simulink model "Block_Diagram_SimulinkNo1"  (R2023b)
settings: Solver=VariableStepAuto  StartTime=0.0  StopTime=20  RelTol=1e-3
values from neighbouring files (symbols this model uses):
  G1_den = [1 0 0]    [Block_DiagramNo1.m]    (also in Block_DiagramNo2.m; CSE_Block_DiagramNo2.m)
  G1_num = [0 0 1]    [Block_DiagramNo1.m]    (also in Block_DiagramNo2.m = [0 1]; CSE_Block_DiagramNo2.m = [0 1])
  G2_den = [1 1]    [Block_DiagramNo1.m]    (also in Block_DiagramNo2.m; CSE_Block_DiagramNo2.m)
  G2_num = [0 0 1]    [Block_DiagramNo1.m]    (also in Block_DiagramNo2.m = [0 1]; CSE_Block_DiagramNo2.m = [0 1])
  G3_den = [1 0]    [Block_DiagramNo1.m]    (also in Block_DiagramNo2.m; CSE_Block_DiagramNo2.m)
  G3_num = [0 1]    [Block_DiagramNo1.m]    (also in Block_DiagramNo2.m; CSE_Block_DiagramNo2.m)
  H1_den = [1 0]    [Block_DiagramNo1.m]    (also in Block_DiagramNo2.m; CSE_Block_DiagramNo2.m)
  H1_num = [0 1]    [Block_DiagramNo1.m]    (also in Block_DiagramNo2.m; CSE_Block_DiagramNo2.m)
  H2_den = [1 -1]    [Block_DiagramNo1.m]    (also in Block_DiagramNo2.m; CSE_Block_DiagramNo2.m)
  H2_num = [0 1]    [Block_DiagramNo1.m]    (also in Block_DiagramNo2.m; CSE_Block_DiagramNo2.m)
  H3_den = [1 -2]    [Block_DiagramNo1.m]    (also in Block_DiagramNo2.m; CSE_Block_DiagramNo2.m)
  H3_num = [0 1]    [Block_DiagramNo1.m]    (also in Block_DiagramNo2.m; CSE_Block_DiagramNo2.m)
  TF_reduced_den = conv(A_den,B_den)    [Block_DiagramNo1.m]
  TF_reduced_num = conv(A_num,B_num)    [Block_DiagramNo1.m]
settings Model: Creator=User  LastModifiedBy=stnlm
settings SolverCC: AlgebraicLoopSolver=TrustRegion
settings DebuggingCC: UnconnectedInputMsg=warning  UnconnectedOutputMsg=warning  UnconnectedLineMsg=warning
settings ModelReferenceCC: EnableRefExpFcnMdlSchedulingChecks=on
settings SFSimCC: CustomCodeUndefinedFunction=UseInterfaceOnly

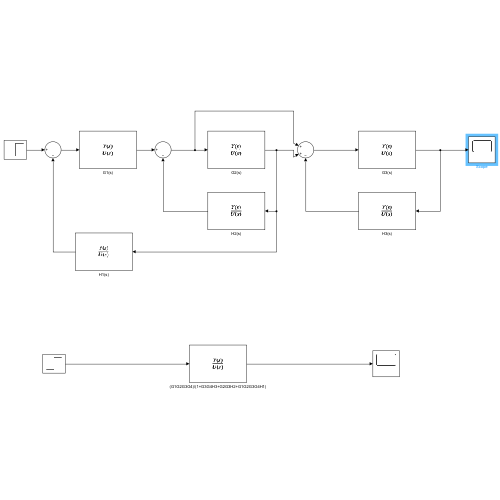
[thumbnail: Simulink's stored preview of the top-level diagram]
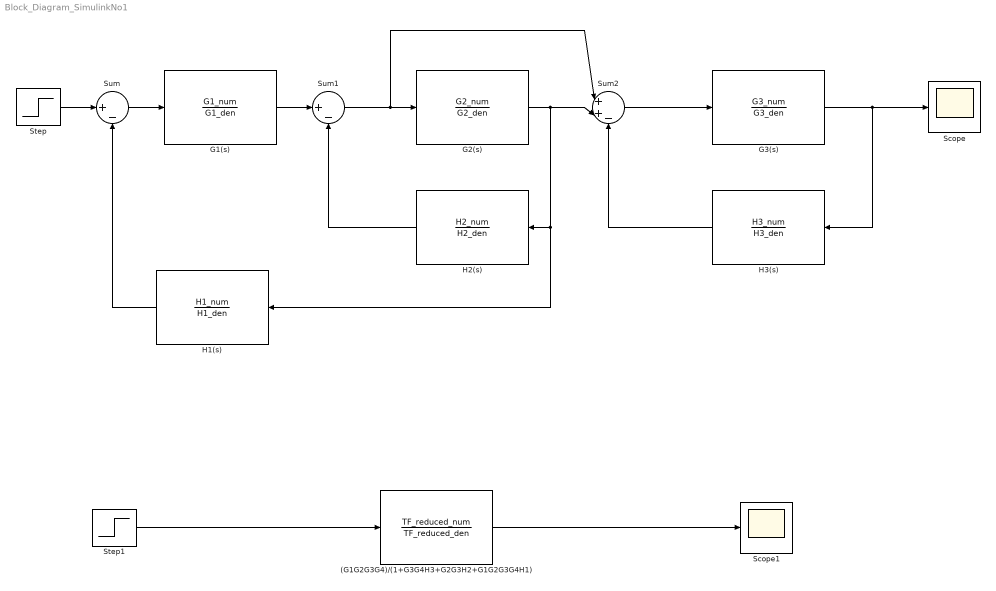
== system Block_Diagram_SimulinkNo1 ==
  (G1G2G3G4)/(1+G3G4H3+G2G3H2+G1G2G3G4H1) : TransferFcn  Numerator=TF_reduced_num  Denominator=TF_reduced_den
  G1(s) : TransferFcn  Numerator=G1_num  Denominator=G1_den
  G2(s) : TransferFcn  Numerator=G2_num  Denominator=G2_den
  G3(s) : TransferFcn  Numerator=G3_num  Denominator=G3_den
  H1(s) : TransferFcn  Numerator=H1_num  Denominator=H1_den
  H2(s) : TransferFcn  Numerator=H2_num  Denominator=H2_den
  H3(s) : TransferFcn  Numerator=H3_num  Denominator=H3_den
  Scope : Scope
  Scope1 : Scope
  Step : Step  SampleTime=0
  Step1 : Step  SampleTime=0
  Sum : Sum  Inputs=|+-
  Sum1 : Sum  Inputs=|+-
  Sum2 : Sum  Inputs=|++-
  wires:
  Step/1 -> Sum/1
  Sum/1 -> G1(s)/1
  G1(s)/1 -> Sum1/1
  H1(s)/1 -> Sum/2
  Sum1/1 -> Sum2/1, G2(s)/1
  G2(s)/1 -> H1(s)/1, H2(s)/1, Sum2/2
  Sum2/1 -> G3(s)/1
  G3(s)/1 -> H3(s)/1, Scope/1
  H2(s)/1 -> Sum1/2
  H3(s)/1 -> Sum2/3
  Step1/1 -> (G1G2G3G4)/(1+G3G4H3+G2G3H2+G1G2G3G4H1)/1
  (G1G2G3G4)/(1+G3G4H3+G2G3H2+G1G2G3G4H1)/1 -> Scope1/1
